simulink model "model"  (R2023a)
settings: Solver=FixedStepAuto  StartTime=0.0  StopTime=5400  FixedStep=0.01  RelTol=1e-3
values from neighbouring files (symbols this model uses):
  A_bhp = area_cilinder    (= 0.006647610055)    [main.m]
  A_bhp_air = A_thp_air    (= 0.0028902652413)    [main.m]
  A_bi = area_cilinder    (= 0.006647610055)    [main.m]
  A_bi_air = A_ti_air    (= 0.00578053048261)    [main.m]
  A_bm = area_cilinder    (= 0.006647610055)    [main.m]
  A_bm_air = A_tm_air    (= 0.0101159283446)    [main.m]
  A_r_air = pi*diam_ring_outer*h_r + 2 * area_ring_outer - area_cilinder    (= 0.0195721222319)    [main.m]
  A_r_tm = pi*diameter_cilinder*h_r_tm    (= 0.00419088459989)    [main.m]
  A_thp = area_cilinder    (= 0.006647610055)    [main.m]
  A_thp_air = pi*diameter_cilinder*d_thp    (= 0.0028902652413)    [main.m]
  A_ti = area_cilinder    (= 0.006647610055)    [main.m]
  A_ti_air = pi*diameter_cilinder*d_ti    (= 0.00578053048261)    [main.m]
  A_tm = area_cilinder    (= 0.006647610055)    [main.m]
  A_tm_air = pi*diameter_cilinder*d_tm    (= 0.0101159283446)    [main.m]
  c_bc = c_tc    (= 460)    [main.m]
  c_bhp = c_tm    (= 460)    [main.m]
  c_bi = c_ti    (= 880)    [main.m]
  c_bm = c_tm    (= 460)    [main.m]
  c_r = 470    [main.m]
  c_tc = c_tm    (= 460)    [main.m]
  c_thp = c_tm    (= 460)    [main.m]
  c_ti = 880    [main.m]
  c_tm = 460    [main.m]
  d_bhp = d_thp    (= 0.01)    [main.m]
  d_bi = d_ti    (= 0.02)    [main.m]
  d_bm = d_tm    (= 0.035)    [main.m]
  d_r = 0.0075    [main.m]
  d_thp = 0.01    [main.m]
  d_ti = 0.02    [main.m]
  d_tm = 0.035    [main.m]
  h_c_bot = 26.5    [main.m]
  h_c_top = h_c_list(i)    [main.m]
  k_bhp = k_tm    (= 22)    [main.m]
  k_bi = k_ti    (= 0.3)    [main.m]
  k_bm = k_tm    (= 22)    [main.m]
  k_r = 22.8    [main.m]
  k_thp = k_tm    (= 22)    [main.m]
  k_ti = 0.3    [main.m]
  k_tm = 22    [main.m]
  m_bc = m_tc    (= 0.0640332)    [main.m]
  m_bhp = m_thp    (= 0.511865974235)    [main.m]
  m_bi = m_ti    (= 0.29249484242)    [main.m]
  m_bm = m_tm    (= 1.79153090982)    [main.m]
  m_r = area_ring_outer*h_r*density_r-area_cilinder*h_r*density_r    (= 0.44801742324)    [main.m]
  m_tc = w_c*h_c*length_c*density_c    (= 0.0640332)    [main.m]
  m_thp = area_cilinder*d_thp*density_m    (= 0.511865974235)    [main.m]
  m_ti = area_cilinder*d_ti*density_i    (= 0.29249484242)    [main.m]
  m_tm = area_cilinder*d_tm*density_m    (= 1.79153090982)    [main.m]
  T_a = 18    [main.m]
  T_init = T_a    (= 18)    [main.m]
settings Model: PauseTimes=2000  Creator=DLubbers  LastModifiedBy=DLubbers
settings OptimizationCC: ReuseModelBlockBuffer=off

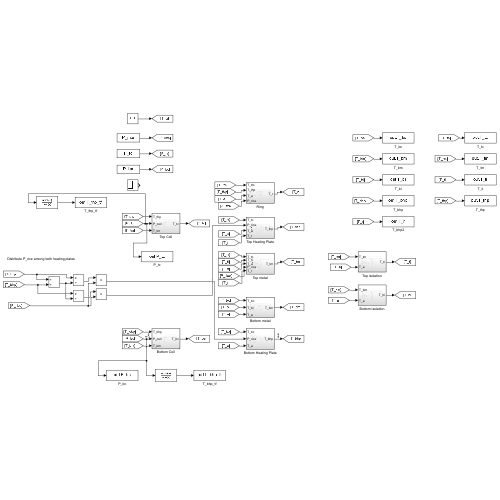
[thumbnail: Simulink's stored preview of the top-level diagram]
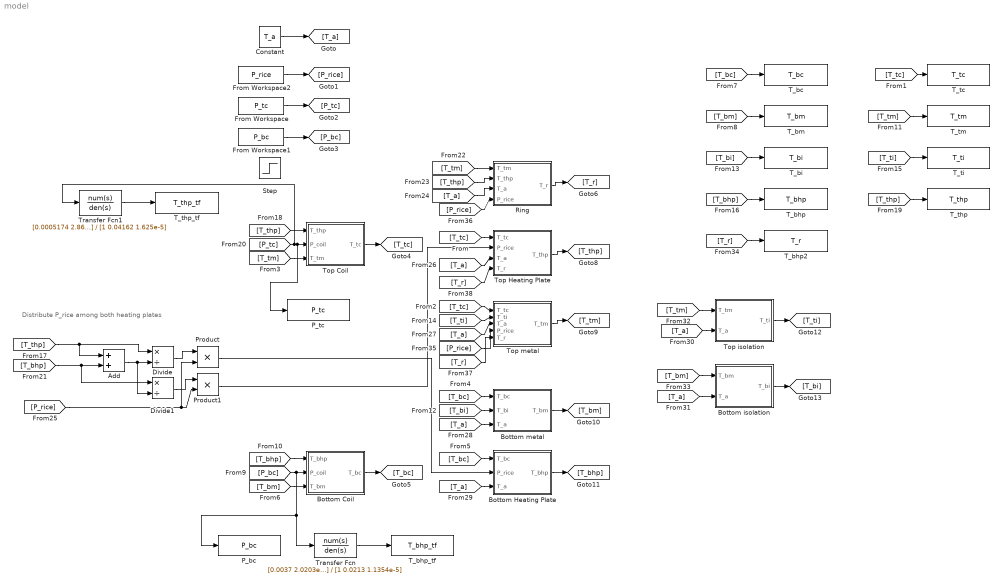
== system model ==
  note: Distribute P_rice among both heating plates
  Add : Sum
  Bottom Coil : Subsystem
  Bottom Heating Plate : Subsystem
  Bottom isolation : Subsystem
  Bottom metal : Subsystem
  Constant : Constant  Value=T_a
  Divide : Product  Inputs=*/
  Divide1 : Product  Inputs=*/
  From Workspace : FromWorkspace  VariableName=P_tc
  From Workspace1 : FromWorkspace  VariableName=P_bc
  From Workspace2 : FromWorkspace  VariableName=P_rice
  P_bc : ToWorkspace  VariableName=P_bc  SaveFormat=Timeseries  SampleTime=-1
  P_tc : ToWorkspace  VariableName=P_tc  SaveFormat=Timeseries  SampleTime=-1
  Product : Product
  Product1 : Product
  Ring : Subsystem
  Step : Step  After=150  SampleTime=0
  T_bc : ToWorkspace  VariableName=T_bc  SaveFormat=Timeseries  SampleTime=-1
  T_bhp : ToWorkspace  VariableName=T_bhp  SaveFormat=Timeseries  SampleTime=-1
  T_bhp2 : ToWorkspace  VariableName=T_r  SaveFormat=Timeseries  SampleTime=-1
  T_bhp_tf : ToWorkspace  VariableName=T_bhp_tf  SaveFormat=Timeseries  SampleTime=-1
  T_bi : ToWorkspace  VariableName=T_bi  SaveFormat=Timeseries  SampleTime=-1
  T_bm : ToWorkspace  VariableName=T_bm  SaveFormat=Timeseries  SampleTime=-1
  T_tc : ToWorkspace  VariableName=T_tc  SaveFormat=Timeseries  SampleTime=-1
  T_thp : ToWorkspace  VariableName=T_thp  SaveFormat=Timeseries  SampleTime=-1
  T_thp_tf : ToWorkspace  VariableName=T_thp_tf  SaveFormat=Timeseries  SampleTime=-1
  T_ti : ToWorkspace  VariableName=T_ti  SaveFormat=Timeseries  SampleTime=-1
  T_tm : ToWorkspace  VariableName=T_tm  SaveFormat=Timeseries  SampleTime=-1
  Top Coil : Subsystem
  Top Heating Plate : Subsystem
  Top isolation : Subsystem
  Top metal : Subsystem
  Transfer Fcn : TransferFcn  Numerator=[0.0037 2.0203e-5]  Denominator=[1 0.0213 1.1354e-5]
  Transfer Fcn1 : TransferFcn  Numerator=[0.0005174 2.864e-5]  Denominator=[1 0.04162 1.625e-5]
  wires:
  Constant/1 -> [T_a]
  From Workspace2/1 -> [P_rice]
  Top Coil/1(T_tc) -> [T_tc]
  Top Heating Plate/1(T_thp) -> [T_thp]
  Top metal/1(T_tm) -> [T_tm]
  Bottom metal/1(T_bm) -> [T_bm]
  Bottom Heating Plate/1(T_bhp) -> [T_bhp]
  Top isolation/1(T_ti) -> [T_ti]
  Bottom isolation/1(T_bi) -> [T_bi]
  [T_tc] -> Top Heating Plate/1(T_tc)
  [T_tc] -> T_tc/1
  [T_tc] -> Top metal/1(T_tc)
  [T_bc] -> Bottom metal/1(T_bc)
  [T_bc] -> Bottom Heating Plate/1(T_bc)
  [T_bc] -> T_bc/1
  [T_bm] -> T_bm/1
  [T_tm] -> T_tm/1
  [T_bi] -> Bottom metal/2(T_bi)
  [T_bi] -> T_bi/1
  [T_ti] -> Top metal/2(T_ti)
  [T_ti] -> T_ti/1
  [T_bhp] -> T_bhp/1
  [T_thp] -> Top Coil/1(T_thp)
  [T_thp] -> T_thp/1
  [P_tc] -> Transfer Fcn1/1, P_tc/1, Top Coil/2(P_coil)
  [T_a] -> Top Heating Plate/3(T_a)
  [T_a] -> Top metal/3(T_a)
  [T_a] -> Bottom metal/3(T_a)
  [T_a] -> Bottom Heating Plate/3(T_a)
  [T_a] -> Top isolation/2(T_a)
  [T_a] -> Bottom isolation/2(T_a)
  [T_tm] -> Top isolation/1(T_tm)
  [T_bm] -> Bottom isolation/1(T_bm)
  [T_tm] -> Top Coil/3(T_tm)
  [T_bm] -> Bottom Coil/3(T_bm)
  [T_bhp] -> Bottom Coil/1(T_bhp)
  Bottom Coil/1(T_bc) -> [T_bc]
  Transfer Fcn/1 -> T_bhp_tf/1
  [P_bc] -> P_bc/1, Transfer Fcn/1, Bottom Coil/2(P_coil)
  [T_tm] -> Ring/1(T_tm)
  [T_thp] -> Ring/2(T_thp)
  [T_a] -> Ring/3(T_a)
  Ring/1(T_r) -> [T_r]
  [T_r] -> T_bhp2/1
  [T_r] -> Top Heating Plate/4(T_r)
  [T_thp] -> Divide/1, Add/1
  [T_bhp] -> Divide1/1, Add/2
  [P_rice] -> Product/2, Product1/2
  [P_rice] -> Top metal/4(P_rice)
  [T_r] -> Top metal/5(T_r)
  Add/1 -> Divide1/2, Divide/2
  Divide/1 -> Product/1
  Divide1/1 -> Product1/1
  Product/1 -> Bottom Heating Plate/2(P_rice)
  Product1/1 -> Top Heating Plate/2(P_rice)
  [P_rice] -> Ring/4(P_rice)
  Transfer Fcn1/1 -> T_thp_tf/1
  From Workspace1/1 -> [P_bc]
  From Workspace/1 -> [P_tc]

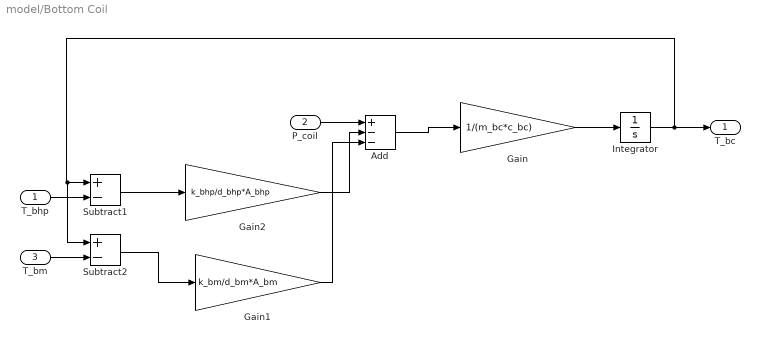
== system model/Bottom Coil ==
  T_bhp : Inport
  P_coil : Inport  Port=2
  T_bm : Inport  Port=3
  Add : Sum  Inputs=+--
  Gain : Gain  Gain=1/(m_bc*c_bc)
  Gain1 : Gain  Gain=k_bm/d_bm*A_bm
  Gain2 : Gain  Gain=k_bhp/d_bhp*A_bhp
  Integrator : Integrator  InitialCondition=T_init
  Subtract1 : Sum  Inputs=+-
  Subtract2 : Sum  Inputs=+-
  T_bc : Outport
  wires:
  Gain/1 -> Integrator/1
  Add/1 -> Gain/1
  Subtract1/1 -> Gain2/1
  Gain2/1 -> Add/2
  T_bhp/1 -> Subtract1/2
  Integrator/1 -> T_bc/1, Subtract2/1, Subtract1/1
  P_coil/1 -> Add/1
  T_bm/1 -> Subtract2/2
  Subtract2/1 -> Gain1/1
  Gain1/1 -> Add/3

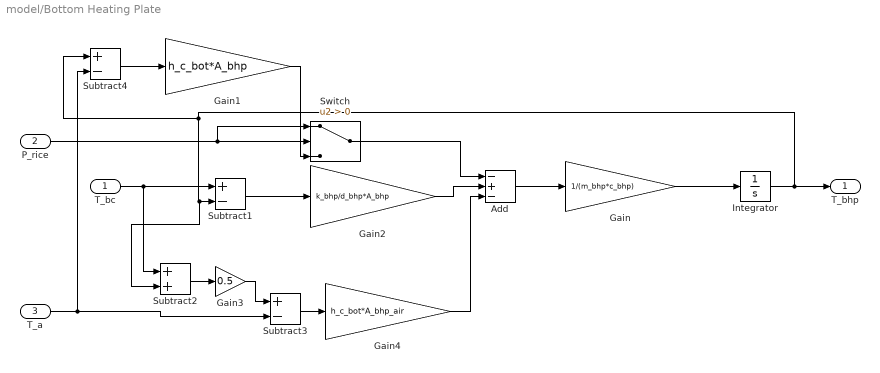
== system model/Bottom Heating Plate ==
  T_bc : Inport
  P_rice : Inport  Port=2
  T_a : Inport  Port=3
  Add : Sum  Inputs=-+-
  Gain : Gain  Gain=1/(m_bhp*c_bhp)
  Gain1 : Gain  Gain=h_c_bot*A_bhp
  Gain2 : Gain  Gain=k_bhp/d_bhp*A_bhp
  Gain3 : Gain  Gain=0.5
  Gain4 : Gain  Gain=h_c_bot*A_bhp_air
  Integrator : Integrator  InitialCondition=T_init
  Subtract1 : Sum  Inputs=+-
  Subtract2 : Sum
  Subtract3 : Sum  Inputs=+-
  Subtract4 : Sum  Inputs=+-
  Switch : Switch  Criteria=u2 > Threshold  SaturateOnIntegerOverflow=off  InputSameDT=off
  T_bhp : Outport
  wires:
  P_rice/1 -> Switch/1, Switch/2
  Gain/1 -> Integrator/1
  Integrator/1 -> T_bhp/1, Subtract4/1, Subtract2/2, Subtract1/2
  Add/1 -> Gain/1
  Subtract1/1 -> Gain2/1
  T_bc/1 -> Subtract2/1, Subtract1/1
  Subtract3/1 -> Gain4/1
  T_a/1 -> Subtract4/2, Subtract3/2
  Subtract2/1 -> Gain3/1
  Gain3/1 -> Subtract3/1
  Gain2/1 -> Add/2
  Gain4/1 -> Add/3
  Switch/1 -> Add/1
  Gain1/1 -> Switch/3
  Subtract4/1 -> Gain1/1

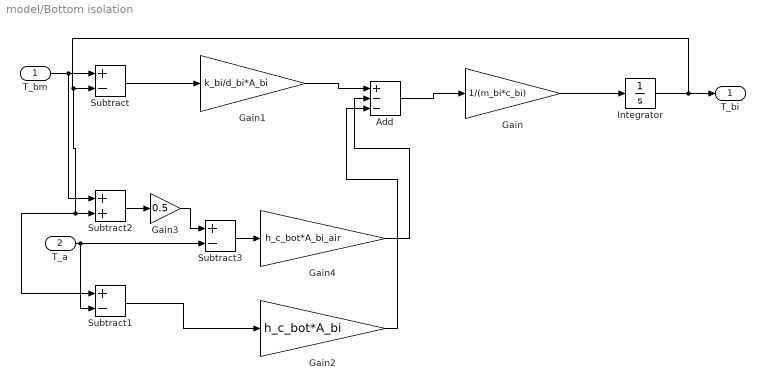
== system model/Bottom isolation ==
  T_bm : Inport
  T_a : Inport  Port=2
  Add : Sum  Inputs=+--
  Gain : Gain  Gain=1/(m_bi*c_bi)
  Gain1 : Gain  Gain=k_bi/d_bi*A_bi
  Gain2 : Gain  Gain=h_c_bot*A_bi
  Gain3 : Gain  Gain=0.5
  Gain4 : Gain  Gain=h_c_bot*A_bi_air
  Integrator : Integrator  InitialCondition=T_init
  Subtract : Sum  Inputs=+-
  Subtract1 : Sum  Inputs=+-
  Subtract2 : Sum
  Subtract3 : Sum  Inputs=+-
  T_bi : Outport
  wires:
  Subtract/1 -> Gain1/1
  Gain/1 -> Integrator/1
  Add/1 -> Gain/1
  Integrator/1 -> Subtract2/2, Subtract1/1, Subtract/2, T_bi/1
  T_bm/1 -> Subtract2/1, Subtract/1
  Gain1/1 -> Add/1
  Subtract2/1 -> Gain3/1
  Gain3/1 -> Subtract3/1
  T_a/1 -> Subtract1/2, Subtract3/2
  Subtract3/1 -> Gain4/1
  Gain4/1 -> Add/2
  Gain2/1 -> Add/3
  Subtract1/1 -> Gain2/1

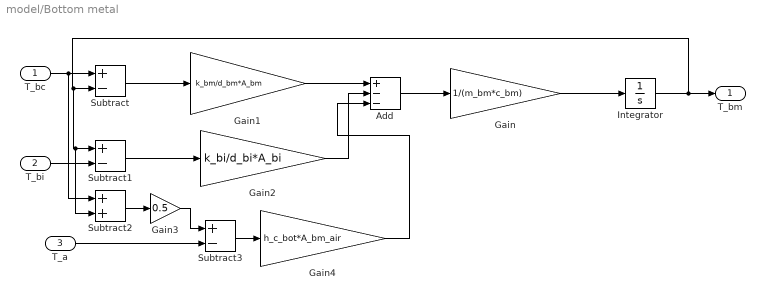
== system model/Bottom metal ==
  T_bc : Inport
  T_bi : Inport  Port=2
  T_a : Inport  Port=3
  Add : Sum  Inputs=+--
  Gain : Gain  Gain=1/(m_bm*c_bm)
  Gain1 : Gain  Gain=k_bm/d_bm*A_bm
  Gain2 : Gain  Gain=k_bi/d_bi*A_bi
  Gain3 : Gain  Gain=0.5
  Gain4 : Gain  Gain=h_c_bot*A_bm_air
  Integrator : Integrator  InitialCondition=T_init
  Subtract : Sum  Inputs=+-
  Subtract1 : Sum  Inputs=+-
  Subtract2 : Sum
  Subtract3 : Sum  Inputs=+-
  T_bm : Outport
  wires:
  Subtract/1 -> Gain1/1
  Gain/1 -> Integrator/1
  Add/1 -> Gain/1
  Subtract1/1 -> Gain2/1
  T_bi/1 -> Subtract1/2
  Integrator/1 -> Subtract2/2, Subtract1/1, Subtract/2, T_bm/1
  T_bc/1 -> Subtract2/1, Subtract/1
  Gain1/1 -> Add/1
  Gain2/1 -> Add/2
  Subtract2/1 -> Gain3/1
  Gain3/1 -> Subtract3/1
  T_a/1 -> Subtract3/2
  Subtract3/1 -> Gain4/1
  Gain4/1 -> Add/3

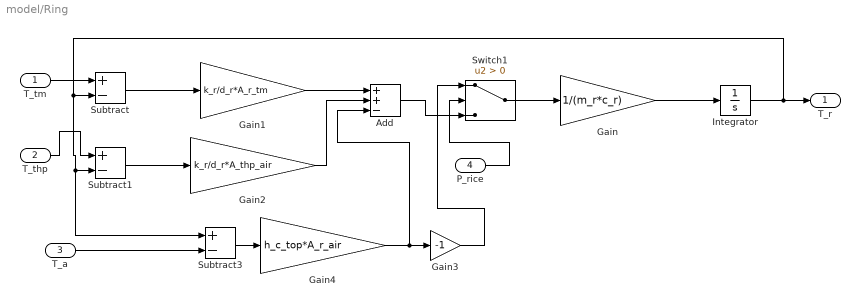
== system model/Ring ==
  T_tm : Inport
  T_thp : Inport  Port=2
  T_a : Inport  Port=3
  P_rice : Inport  Port=4
  Add : Sum  Inputs=++-
  Gain : Gain  Gain=1/(m_r*c_r)
  Gain1 : Gain  Gain=k_r/d_r*A_r_tm
  Gain2 : Gain  Gain=k_r/d_r*A_thp_air
  Gain3 : Gain  Gain=-1
  Gain4 : Gain  Gain=h_c_top*A_r_air
  Integrator : Integrator  InitialCondition=T_init
  Subtract : Sum  Inputs=+-
  Subtract1 : Sum  Inputs=+-
  Subtract3 : Sum  Inputs=+-
  Switch1 : Switch  Criteria=u2 > Threshold  SaturateOnIntegerOverflow=off  InputSameDT=off
  T_r : Outport
  wires:
  Subtract/1 -> Gain1/1
  Gain/1 -> Integrator/1
  Subtract1/1 -> Gain2/1
  Integrator/1 -> Subtract3/1, Subtract1/2, Subtract/2, T_r/1
  T_tm/1 -> Subtract/1
  Gain1/1 -> Add/1
  Gain2/1 -> Add/2
  T_a/1 -> Subtract3/2
  Subtract3/1 -> Gain4/1
  T_thp/1 -> Subtract1/1
  P_rice/1 -> Switch1/2
  Switch1/1 -> Gain/1
  Add/1 -> Switch1/3
  Gain4/1 -> Gain3/1, Add/3
  Gain3/1 -> Switch1/1

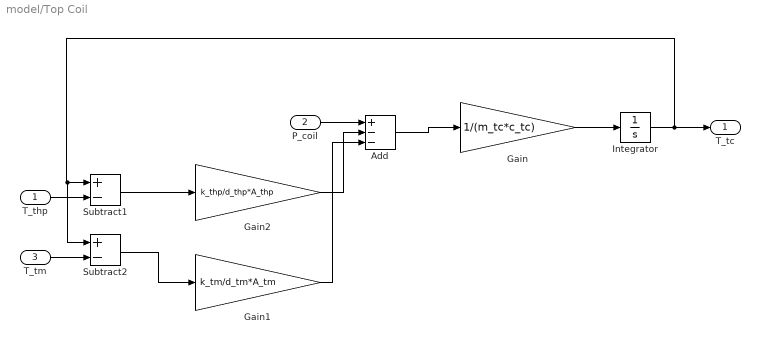
== system model/Top Coil ==
  T_thp : Inport
  P_coil : Inport  Port=2
  T_tm : Inport  Port=3
  Add : Sum  Inputs=+--
  Gain : Gain  Gain=1/(m_tc*c_tc)
  Gain1 : Gain  Gain=k_tm/d_tm*A_tm
  Gain2 : Gain  Gain=k_thp/d_thp*A_thp
  Integrator : Integrator  InitialCondition=T_init
  Subtract1 : Sum  Inputs=+-
  Subtract2 : Sum  Inputs=+-
  T_tc : Outport
  wires:
  Gain/1 -> Integrator/1
  Add/1 -> Gain/1
  Subtract1/1 -> Gain2/1
  Gain2/1 -> Add/2
  T_thp/1 -> Subtract1/2
  Integrator/1 -> T_tc/1, Subtract2/1, Subtract1/1
  P_coil/1 -> Add/1
  T_tm/1 -> Subtract2/2
  Subtract2/1 -> Gain1/1
  Gain1/1 -> Add/3

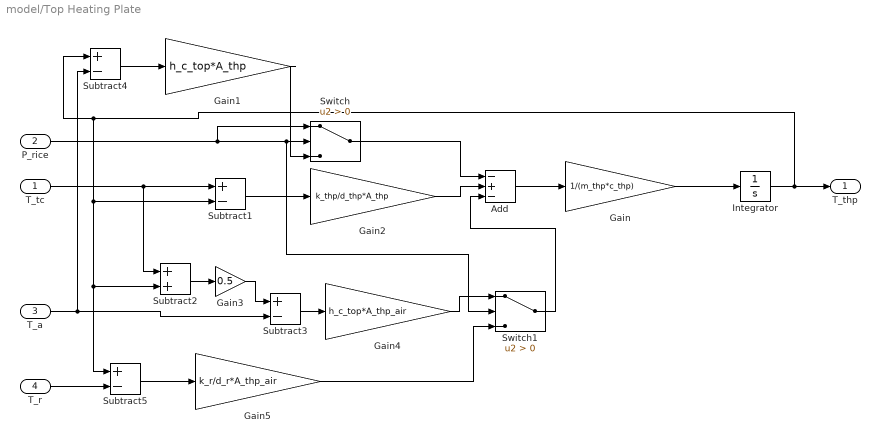
== system model/Top Heating Plate ==
  T_tc : Inport
  P_rice : Inport  Port=2
  T_a : Inport  Port=3
  T_r : Inport  Port=4
  Add : Sum  Inputs=-+-
  Gain : Gain  Gain=1/(m_thp*c_thp)
  Gain1 : Gain  Gain=h_c_top*A_thp
  Gain2 : Gain  Gain=k_thp/d_thp*A_thp
  Gain3 : Gain  Gain=0.5
  Gain4 : Gain  Gain=h_c_top*A_thp_air
  Gain5 : Gain  Gain=k_r/d_r*A_thp_air
  Integrator : Integrator  InitialCondition=T_init
  Subtract{1,3..5} (4 alike) : Sum  Inputs=+-
  Subtract2 : Sum
  Switch : Switch  Criteria=u2 > Threshold  SaturateOnIntegerOverflow=off  InputSameDT=off
  Switch1 : Switch  Criteria=u2 > Threshold  SaturateOnIntegerOverflow=off  InputSameDT=off
  T_thp : Outport
  wires:
  P_rice/1 -> Switch/1, Switch1/2, Switch/2
  Gain/1 -> Integrator/1
  Integrator/1 -> T_thp/1, Subtract4/1, Subtract1/2, Subtract2/2, Subtract5/1
  Add/1 -> Gain/1
  Subtract1/1 -> Gain2/1
  T_tc/1 -> Subtract2/1, Subtract1/1
  Subtract3/1 -> Gain4/1
  T_a/1 -> Subtract4/2, Subtract3/2
  Subtract2/1 -> Gain3/1
  Gain3/1 -> Subtract3/1
  Gain2/1 -> Add/2
  Switch/1 -> Add/1
  Gain1/1 -> Switch/3
  Subtract4/1 -> Gain1/1
  T_r/1 -> Subtract5/2
  Subtract5/1 -> Gain5/1
  Gain4/1 -> Switch1/1
  Gain5/1 -> Switch1/3
  Switch1/1 -> Add/3

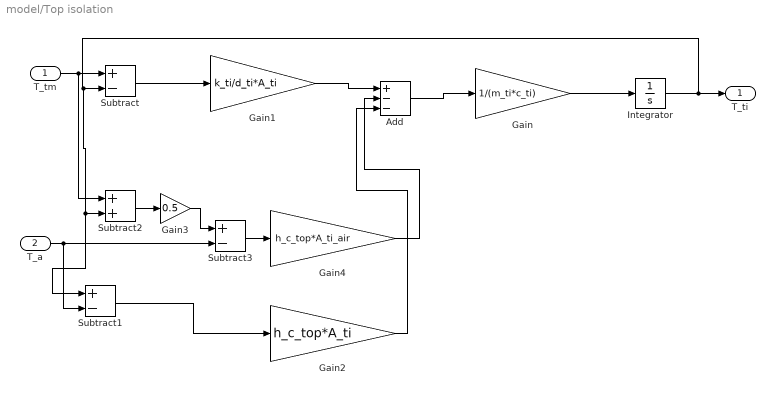
== system model/Top isolation ==
  T_tm : Inport
  T_a : Inport  Port=2
  Add : Sum  Inputs=+--
  Gain : Gain  Gain=1/(m_ti*c_ti)
  Gain1 : Gain  Gain=k_ti/d_ti*A_ti
  Gain2 : Gain  Gain=h_c_top*A_ti
  Gain3 : Gain  Gain=0.5
  Gain4 : Gain  Gain=h_c_top*A_ti_air
  Integrator : Integrator  InitialCondition=T_init
  Subtract : Sum  Inputs=+-
  Subtract1 : Sum  Inputs=+-
  Subtract2 : Sum
  Subtract3 : Sum  Inputs=+-
  T_ti : Outport
  wires:
  Subtract/1 -> Gain1/1
  Gain/1 -> Integrator/1
  Add/1 -> Gain/1
  Integrator/1 -> Subtract1/1, Subtract2/2, Subtract/2, T_ti/1
  T_tm/1 -> Subtract2/1, Subtract/1
  Gain1/1 -> Add/1
  Subtract2/1 -> Gain3/1
  Gain3/1 -> Subtract3/1
  T_a/1 -> Subtract1/2, Subtract3/2
  Subtract3/1 -> Gain4/1
  Gain4/1 -> Add/2
  Gain2/1 -> Add/3
  Subtract1/1 -> Gain2/1

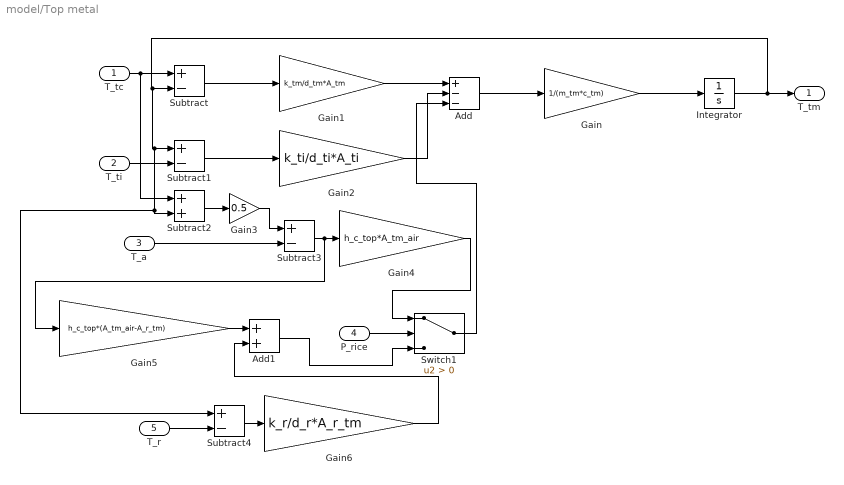
== system model/Top metal ==
  T_tc : Inport
  T_ti : Inport  Port=2
  T_a : Inport  Port=3
  P_rice : Inport  Port=4
  T_r : Inport  Port=5
  Add : Sum  Inputs=+--
  Add1 : Sum
  Gain : Gain  Gain=1/(m_tm*c_tm)
  Gain1 : Gain  Gain=k_tm/d_tm*A_tm
  Gain2 : Gain  Gain=k_ti/d_ti*A_ti
  Gain3 : Gain  Gain=0.5
  Gain4 : Gain  Gain=h_c_top*A_tm_air
  Gain5 : Gain  Gain=h_c_top*(A_tm_air-A_r_tm)
  Gain6 : Gain  Gain=k_r/d_r*A_r_tm
  Integrator : Integrator  InitialCondition=T_init
  Subtract{,1,3..4} (4 alike) : Sum  Inputs=+-
  Subtract2 : Sum
  Switch1 : Switch  Criteria=u2 > Threshold  SaturateOnIntegerOverflow=off  InputSameDT=off
  T_tm : Outport
  wires:
  Subtract/1 -> Gain1/1
  Gain/1 -> Integrator/1
  Add/1 -> Gain/1
  Subtract1/1 -> Gain2/1
  T_ti/1 -> Subtract1/2
  Integrator/1 -> Subtract4/1, Subtract2/2, Subtract1/1, Subtract/2, T_tm/1
  T_tc/1 -> Subtract/1, Subtract2/1
  Gain1/1 -> Add/1
  Gain2/1 -> Add/2
  Subtract2/1 -> Gain3/1
  Gain3/1 -> Subtract3/1
  T_a/1 -> Subtract3/2
  Subtract3/1 -> Gain5/1, Gain4/1
  P_rice/1 -> Switch1/2
  Switch1/1 -> Add/3
  Gain5/1 -> Add1/1
  T_r/1 -> Subtract4/2
  Subtract4/1 -> Gain6/1
  Gain6/1 -> Add1/2
  Add1/1 -> Switch1/3
  Gain4/1 -> Switch1/1
